simulink model "model_regulator3"  (R2024a)
settings: Solver=FixedStepAuto  StartTime=0.0  StopTime=10.0  FixedStep=0.001  RelTol=1e-3
undefined symbols (not defined in the file): k
settings Model: Creator=main  LastModifiedBy=main

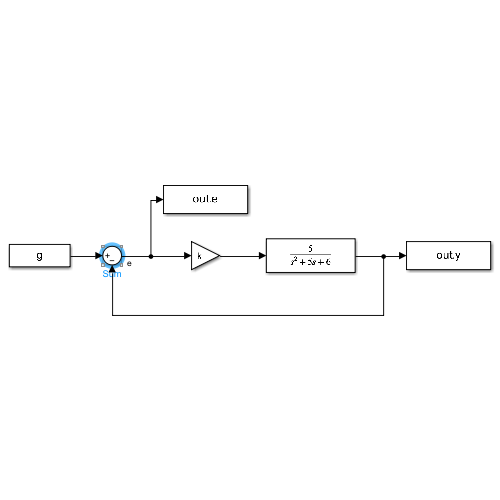
[thumbnail: Simulink's stored preview of the top-level diagram]
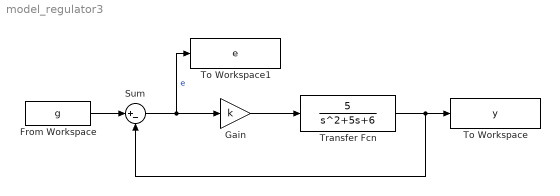
== system model_regulator3 ==
  From Workspace : FromWorkspace  VariableName=g
  Gain : Gain  Gain=k
  Sum : Sum  Inputs=|+-
  To Workspace : ToWorkspace  VariableName=y  SaveFormat=Timeseries  SampleTime=-1
  To Workspace1 : ToWorkspace  VariableName=e  SaveFormat=Timeseries  SampleTime=-1
  Transfer Fcn : TransferFcn  Numerator=[5]  Denominator=[1 5 6]
  wires:
  Transfer Fcn/1 -> Sum/2, To Workspace/1
  From Workspace/1 -> Sum/1
  Gain/1 -> Transfer Fcn/1
  Sum/1 -> To Workspace1/1, Gain/1  "e"
